simulink model "Adaptive_Cruise_Control_Logic"  (R2021a)
settings: Solver=FixedStepDiscrete  StartTime=0.0  StopTime=10.0  FixedStep=0.01  RelTol=1e-3
settings Model: DataDictionary=ACC_SLDD.sldd  Creator=Gaurav  LastModifiedBy=Gaurav
settings OptimizationCC: DefaultParameterBehavior=Inlined  EnhancedBackFolding=on  PassReuseOutputArgsAs=Individual arguments  ZeroExternalMemoryAtStartup=off  ZeroInternalMemoryAtStartup=off  OptimizeBlockOrder=speed  DifferentSizesBufferReuse=on  OptimizationCustomize=off  EfficientTunableParamExpr=on
settings DebuggingCC: SignalInfNanChecking=error  CheckMatrixSingularityMsg=error  IntegerOverflowMsg=error  ParameterTunabilityLossMsg=error  UniqueDataStoreMsg=warning  StrictBusMsg=ErrorOnBusTreatedAsVector  IntegerSaturationMsg=error
settings SFSimCC: MATLABDynamicMemAlloc=off
settings RTWCC: SystemTargetFile=ert.tlc  TemplateMakefile=ert_default_tmf
settings CodeAppCC: ForceParamTrailComments=on  IgnoreCustomStorageClasses=off  OperatorAnnotations=on  SimulinkDataObjDesc=on  SFDataObjDesc=on  InsertBlockDesc=on
settings ERTTargetCC: TargetLangStandard=C99 (ISO)  GenerateSampleERTMain=on  InlinedParameterPlacement=NonHierarchical  ERTCustomFileTemplate=example_file_process.tlc
settings ConfigComp: CovEnable=on  RecordCoverage=on  CovMetricSettings=dcmwe  CovModelRefEnable=on

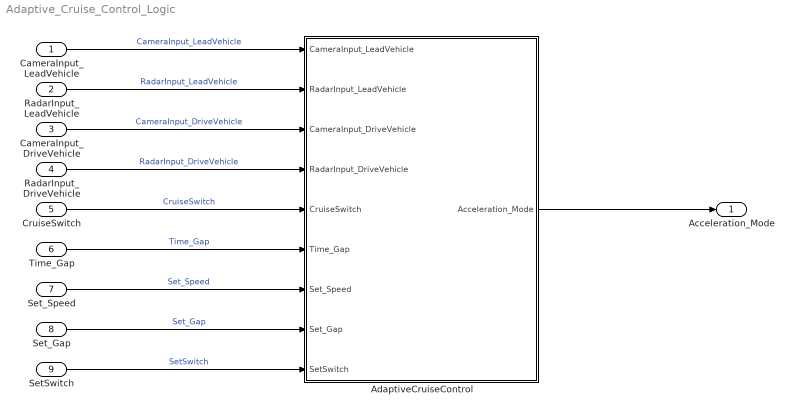
== system Adaptive_Cruise_Control_Logic ==
  CameraInput_LeadVehicle : Inport
  RadarInput_LeadVehicle : Inport  Port=2
  CameraInput_DriveVehicle : Inport  Port=3
  RadarInput_DriveVehicle : Inport  Port=4
  CruiseSwitch : Inport  Port=5
  Time_Gap : Inport  Port=6
  Set_Speed : Inport  Port=7
  Set_Gap : Inport  Port=8
  SetSwitch : Inport  Port=9
  AdaptiveCruiseControl : Subsystem  TreatAsAtomicUnit=on  SystemSampleTime=0.01
  Acceleration_Mode : Outport
  wires:
  CameraInput_DriveVehicle/1 -> AdaptiveCruiseControl/3(CameraInput_DriveVehicle)  "CameraInput_DriveVehicle"
  CruiseSwitch/1 -> AdaptiveCruiseControl/5(CruiseSwitch)  "CruiseSwitch"
  Set_Speed/1 -> AdaptiveCruiseControl/7(Set_Speed)  "Set_Speed"
  AdaptiveCruiseControl/1(Acceleration_Mode) -> Acceleration_Mode/1
  SetSwitch/1 -> AdaptiveCruiseControl/9(SetSwitch)  "SetSwitch"
  Set_Gap/1 -> AdaptiveCruiseControl/8(Set_Gap)  "Set_Gap"
  Time_Gap/1 -> AdaptiveCruiseControl/6(Time_Gap)  "Time_Gap"
  RadarInput_DriveVehicle/1 -> AdaptiveCruiseControl/4(RadarInput_DriveVehicle)  "RadarInput_DriveVehicle"
  RadarInput_LeadVehicle/1 -> AdaptiveCruiseControl/2(RadarInput_LeadVehicle)  "RadarInput_LeadVehicle"
  CameraInput_LeadVehicle/1 -> AdaptiveCruiseControl/1(CameraInput_LeadVehicle)  "CameraInput_LeadVehicle"

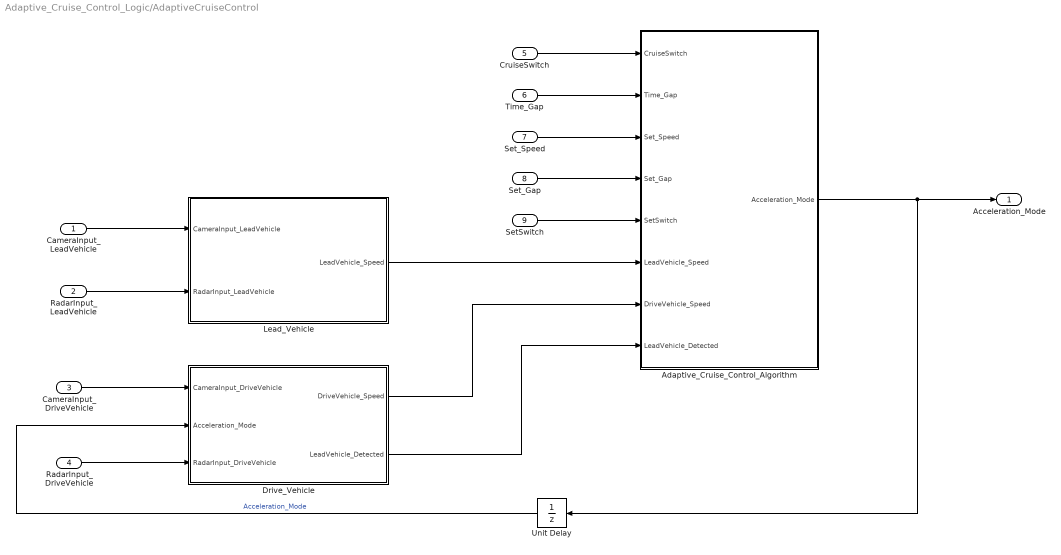
== system Adaptive_Cruise_Control_Logic/AdaptiveCruiseControl ==
  CameraInput_LeadVehicle : Inport
  RadarInput_LeadVehicle : Inport  Port=2
  CameraInput_DriveVehicle : Inport  Port=3
  RadarInput_DriveVehicle : Inport  Port=4
  CruiseSwitch : Inport  Port=5
  Time_Gap : Inport  Port=6
  Set_Speed : Inport  Port=7
  Set_Gap : Inport  Port=8
  SetSwitch : Inport  Port=9
  Adaptive_Cruise_Control_Algorithm : Subsystem
  Drive_Vehicle : Subsystem
  Lead_Vehicle : Subsystem
  Unit Delay : UnitDelay  SampleTime=-1  StateName=Acceleration_Mode  HasFrameUpgradeWarning=on
  Acceleration_Mode : Outport
  wires:
  CameraInput_LeadVehicle/1 -> Lead_Vehicle/1(CameraInput_LeadVehicle)
  RadarInput_LeadVehicle/1 -> Lead_Vehicle/2(RadarInput_LeadVehicle)
  RadarInput_DriveVehicle/1 -> Drive_Vehicle/3(RadarInput_DriveVehicle)
  CameraInput_DriveVehicle/1 -> Drive_Vehicle/1(CameraInput_DriveVehicle)
  Adaptive_Cruise_Control_Algorithm/1(Acceleration_Mode) -> Unit Delay/1, Acceleration_Mode/1
  Drive_Vehicle/2(LeadVehicle_Detected) -> Adaptive_Cruise_Control_Algorithm/8(LeadVehicle_Detected)
  Drive_Vehicle/1(DriveVehicle_Speed) -> Adaptive_Cruise_Control_Algorithm/7(DriveVehicle_Speed)
  Lead_Vehicle/1(LeadVehicle_Speed) -> Adaptive_Cruise_Control_Algorithm/6(LeadVehicle_Speed)
  CruiseSwitch/1 -> Adaptive_Cruise_Control_Algorithm/1(CruiseSwitch)
  Time_Gap/1 -> Adaptive_Cruise_Control_Algorithm/2(Time_Gap)
  Set_Speed/1 -> Adaptive_Cruise_Control_Algorithm/3(Set_Speed)
  Set_Gap/1 -> Adaptive_Cruise_Control_Algorithm/4(Set_Gap)
  SetSwitch/1 -> Adaptive_Cruise_Control_Algorithm/5(SetSwitch)
  Unit Delay/1 -> Drive_Vehicle/2(Acceleration_Mode)  "Acceleration_Mode"

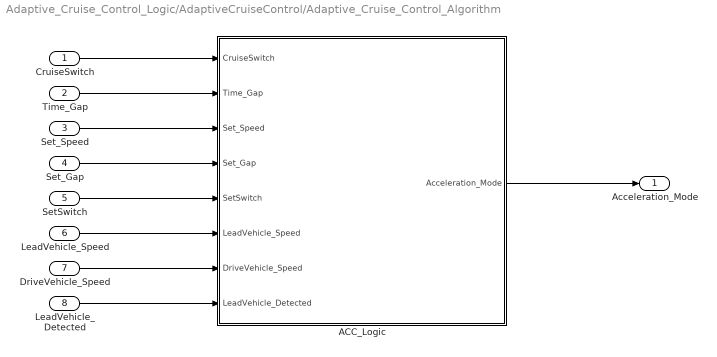
== system Adaptive_Cruise_Control_Logic/AdaptiveCruiseControl/Adaptive_Cruise_Control_Algorithm ==
  CruiseSwitch : Inport
  Time_Gap : Inport  Port=2
  Set_Speed : Inport  Port=3
  Set_Gap : Inport  Port=4
  SetSwitch : Inport  Port=5
  LeadVehicle_Speed : Inport  Port=6
  DriveVehicle_Speed : Inport  Port=7
  LeadVehicle_Detected : Inport  Port=8
  ACC_Logic : Stateflow chart  TreatAsAtomicUnit=on
  Acceleration_Mode : Outport
  wires:
  Set_Gap/1 -> ACC_Logic/4(Set_Gap)
  SetSwitch/1 -> ACC_Logic/5(SetSwitch)
  Time_Gap/1 -> ACC_Logic/2(Time_Gap)
  CruiseSwitch/1 -> ACC_Logic/1(CruiseSwitch)
  Set_Speed/1 -> ACC_Logic/3(Set_Speed)
  LeadVehicle_Speed/1 -> ACC_Logic/6(LeadVehicle_Speed)
  DriveVehicle_Speed/1 -> ACC_Logic/7(DriveVehicle_Speed)
  LeadVehicle_Detected/1 -> ACC_Logic/8(LeadVehicle_Detected)
  ACC_Logic/1(Acceleration_Mode) -> Acceleration_Mode/1

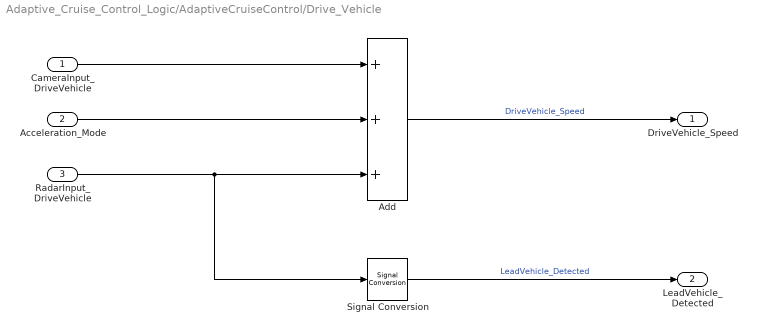
== system Adaptive_Cruise_Control_Logic/AdaptiveCruiseControl/Drive_Vehicle ==
  CameraInput_DriveVehicle : Inport
  Acceleration_Mode : Inport  Port=2
  RadarInput_DriveVehicle : Inport  Port=3
  Add : Sum  Inputs=+++  OutDataTypeStr=Inherit: Inherit via back propagation
  Signal Conversion : SignalConversion  OverrideOpt=off
  DriveVehicle_Speed : Outport
  LeadVehicle_Detected : Outport  Port=2
  wires:
  CameraInput_DriveVehicle/1 -> Add/1
  RadarInput_DriveVehicle/1 -> Signal Conversion/1, Add/3
  Add/1 -> DriveVehicle_Speed/1  "DriveVehicle_Speed"
  Acceleration_Mode/1 -> Add/2
  Signal Conversion/1 -> LeadVehicle_Detected/1  "LeadVehicle_Detected"

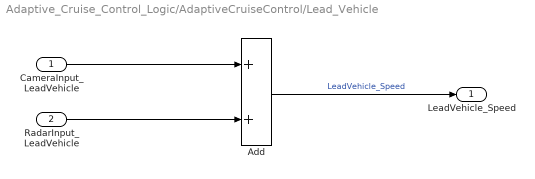
== system Adaptive_Cruise_Control_Logic/AdaptiveCruiseControl/Lead_Vehicle ==
  CameraInput_LeadVehicle : Inport
  RadarInput_LeadVehicle : Inport  Port=2
  Add : Sum  OutDataTypeStr=Inherit: Inherit via back propagation
  LeadVehicle_Speed : Outport
  wires:
  CameraInput_LeadVehicle/1 -> Add/1
  RadarInput_LeadVehicle/1 -> Add/2
  Add/1 -> LeadVehicle_Speed/1  "LeadVehicle_Speed"

== stateflow chart Adaptive_Cruise_Control_Logic/AdaptiveCruiseControl/Adaptive_Cruise_Control_Algorithm/ACC_Logic ==
  state ACC_STANDBY_MODE
    entry:
    Acceleration_Mode=1;
  state ACC_OFF_MODE
    entry:
    Acceleration_Mode = 0;
  state ACC_ON_MODE
    state LeadVehicle_Detected_Resume
      entry:
      Acceleration_Mode=3;
    state LeadVehicle_Not_Detected_Resume
      entry:
      Acceleration_Mode=1;
    state LeadVehicle_Detected_Follow
      entry:
      Acceleration_Mode=2;
    state LeadVehicle_Not_Detected
      entry:
      Acceleration_Mode=1;
    state LeadVehicle_Speed_lessthan_Set_Speed
      entry:
      Acceleration_Mode=4;
    state LeadVehicle_Speed_equal_Set_Speed
      entry:
      Acceleration_Mode=5;
    (default) -> LeadVehicle_Detected_Follow
    LeadVehicle_Detected_Resume -> LeadVehicle_Detected_Follow [order 1] : [(DriveVehicle_Speed == Set_Speed) &&...
        |  (LeadVehicle_Speed >= Set_Speed) &&...
        |  (Time_Gap >= Set_Gap)]
    LeadVehicle_Detected_Resume -> LeadVehicle_Not_Detected_Resume [order 2] : [LeadVehicle_Detected==0]
    LeadVehicle_Detected_Follow -> LeadVehicle_Not_Detected [order 1] : [LeadVehicle_Detected == 0]
    LeadVehicle_Not_Detected -> LeadVehicle_Detected_Follow [order 1] : [(LeadVehicle_Detected == 1)&&...
        | (DriveVehicle_Speed == Set_Speed) &&...
        | (LeadVehicle_Speed >= Set_Speed) &&...
        | (Time_Gap >= Set_Gap)]
    LeadVehicle_Speed_equal_Set_Speed -> LeadVehicle_Detected_Resume [order 1] : [(DriveVehicle_Speed < Set_Speed) &&...
        |  (LeadVehicle_Speed > DriveVehicle_Speed) &&...
        |  (Time_Gap >= Set_Gap)]
    LeadVehicle_Detected_Resume -> LeadVehicle_Speed_equal_Set_Speed [order 3] : [(DriveVehicle_Speed < Set_Speed) &&...
        |  (LeadVehicle_Speed > DriveVehicle_Speed) ||...
        |  (Time_Gap >= Set_Gap)]
    LeadVehicle_Speed_equal_Set_Speed -> LeadVehicle_Not_Detected_Resume [order 2] : [(LeadVehicle_Detected == 0) ||...
        | (DriveVehicle_Speed <= Set_Speed)]
    LeadVehicle_Detected_Follow -> LeadVehicle_Speed_lessthan_Set_Speed [order 2] : [(LeadVehicle_Detected == 1)&&...
        | (DriveVehicle_Speed < Set_Speed) ||...
        | (Time_Gap < Set_Gap)]
    LeadVehicle_Not_Detected -> LeadVehicle_Speed_lessthan_Set_Speed [order 2] : [(LeadVehicle_Detected == 1) &&...
        | (DriveVehicle_Speed < Set_Speed) ||...
        | (Time_Gap < Set_Gap)]
    LeadVehicle_Speed_lessthan_Set_Speed -> LeadVehicle_Not_Detected [order 1] : [(LeadVehicle_Detected == 0) &&...
        | (DriveVehicle_Speed == Set_Speed)]
    LeadVehicle_Speed_equal_Set_Speed -> LeadVehicle_Speed_lessthan_Set_Speed [order 3] : [(LeadVehicle_Speed < Set_Speed) &&...
        | (LeadVehicle_Speed < DriveVehicle_Speed) ||...
        | (Time_Gap ==0.75*Set_Gap)]
    LeadVehicle_Speed_lessthan_Set_Speed -> LeadVehicle_Speed_equal_Set_Speed [order 2] : [((LeadVehicle_Speed*1.25>=DriveVehicle_Speed) &&...
        | (LeadVehicle_Speed * 0.75<=DriveVehicle_Speed)) &&...
        | (DriveVehicle_Speed < Set_Speed) &&...
        | ((Time_Gap<=1.25*Set_Gap) &&...
        | (Time_Gap >=0.75*Set_Gap))]
  (default) -> ACC_OFF_MODE
  ACC_OFF_MODE -> ACC_STANDBY_MODE : [CruiseSwitch==1]
  ACC_STANDBY_MODE -> ACC_OFF_MODE [order 1] : [CruiseSwitch==0]
  ACC_ON_MODE -> ACC_OFF_MODE [order 2] : [CruiseSwitch==0]
  ACC_STANDBY_MODE -> ACC_ON_MODE [order 2] : [SetSwitch==1]
  ACC_ON_MODE -> ACC_STANDBY_MODE [order 1] : [SetSwitch==0]
  data: CruiseSwitch input size=1; Time_Gap input size=1; Set_Speed input size=1; Set_Gap input size=1; SetSwitch input size=1; LeadVehicle_Speed input size=1; DriveVehicle_Speed input size=1; LeadVehicle_Detected input size=1; Acceleration_Mode output uint8 size=1
